simulink model "sim12xxd"  (Simulink 4.00)
settings: Solver=ode45  SolverMode=SingleTasking  StartTime=0.0  StopTime=3  MaxStep=.050  RelTol=1e-3  AbsTol=1e-3
settings Model: LastModifiedBy=saadat  SaveTime=off  SaveOutput=off  LimitDataPoints=off  RTWTemplateMakefile=grt_vc.tmf  ExtModeTrigMode=oneshot  ExtModeArmWhenConnect=off

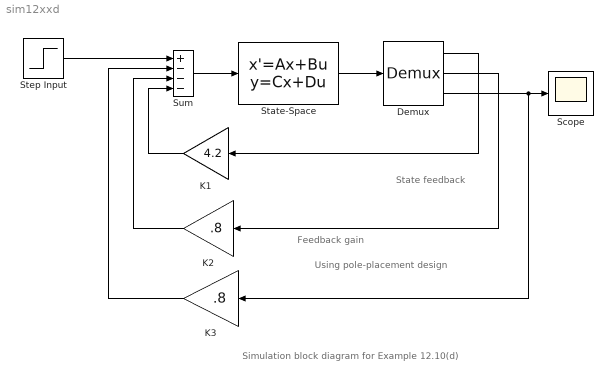
== system sim12xxd ==
  note: Simulation block diagram for Example 12.10(d)
  note: Using pole-placement design
  note: Feedback gain
  note: State feedback
  Demux : Demux  Outputs=3  BusSelectionMode=off
  K1 : Gain  Orientation=left  Gain=4.2  Multiplication=Element-wise(K.*u)  SaturateOnIntegerOverflow=on
  K2 : Gain  Orientation=left  Gain=.8  Multiplication=Element-wise(K.*u)  SaturateOnIntegerOverflow=on
  K3 : Gain  Orientation=left  Gain=.8  Multiplication=Element-wise(K.*u)  SaturateOnIntegerOverflow=on
  Scope : Scope
      settings: TickLabels=on  TimeRange=3  YMin=-0.004  YMax=0  SaveToWorkspace=off  SaveName=ScopeData  DataFormat=Array  LimitDataPoints=on  MaxDataPoints=5000
  State-Space : StateSpace  A="[-5  0  -100;  2  -2  0;  0  0.1  -0.08]"  B="[0;   0 ;  -0.1]"  C=eye(3)  D=zeros(3, 1)  X0=0  AbsoluteTolerance=auto  Realization=auto
  Step Input : Step  Time=0  Before=0  After=0.2  SampleTime=0
  Sum : Sum  Inputs=+---  SaturateOnIntegerOverflow=on
  wires:
  K3/1 -> Sum/2
  Demux/3 -> K3/1, Scope/1
  Step Input/1 -> Sum/1
  K2/1 -> Sum/3
  K1/1 -> Sum/4
  Sum/1 -> State-Space/1
  Demux/2 -> K2/1
  Demux/1 -> K1/1
  State-Space/1 -> Demux/1
